simulink model "LQR"  (R2018a)
settings: Solver=ode45  StartTime=0.0  StopTime=10.0  RelTol=1e-3  EnableMultiTasking=on
values from neighbouring files (symbols this model uses):
  A = input('enter the A matrix = ')    [LQR2.m]
  B = input('enter the B matrix = ')    [LQR2.m]
  Q = transpose(C)*C    [LQR2.m]
  R = input('enter the matrix of R(no. of columns must be equal to B) = ')    [LQR2.m]
undefined symbols (not defined in the file or in its folder): X0
libraries: dspinverses x1
settings Model: Creator=gkavuran  LastModifiedBy=Jay
settings DataIOCC: LimitDataPoints=on  SaveFormat=Array
settings OptimizationCC: LifeSpan=inf
settings DebuggingCC: SolverPrmCheckMsg=warning  SFUnexpectedBacktrackingDiag=warning  SFNoUnconditionalDefaultTransitionDiag=warning  SFExecutionAtInitializationDiag=none
settings HardwareCC: ProdBitPerPointer=32  ProdBitPerSizeT=32  ProdBitPerPtrDiffT=32  ProdLargestAtomicFloat=None  ProdIntDivRoundTo=Undefined  ProdEndianess=Unspecified  ProdWordSize=32  ProdHWDeviceType=32-bit Generic
settings ModelReferenceCC: PropagateSignalLabelsOutOfModel=off
settings CodeAppCC: StateflowObjectComments=on
settings GRTTargetCC: TargetLangStandard=C89/C90 (ANSI)  GeneratePreprocessorConditionals=Disable all
settings ConfigComp: CovMetricSettings=dw  CovHtmlReporting=on  CovSaveCumulativeToWorkspaceVar=on  CovSaveSingleToWorkspaceVar=on  CovExternalEMLEnable=off  CovSFcnEnable=off

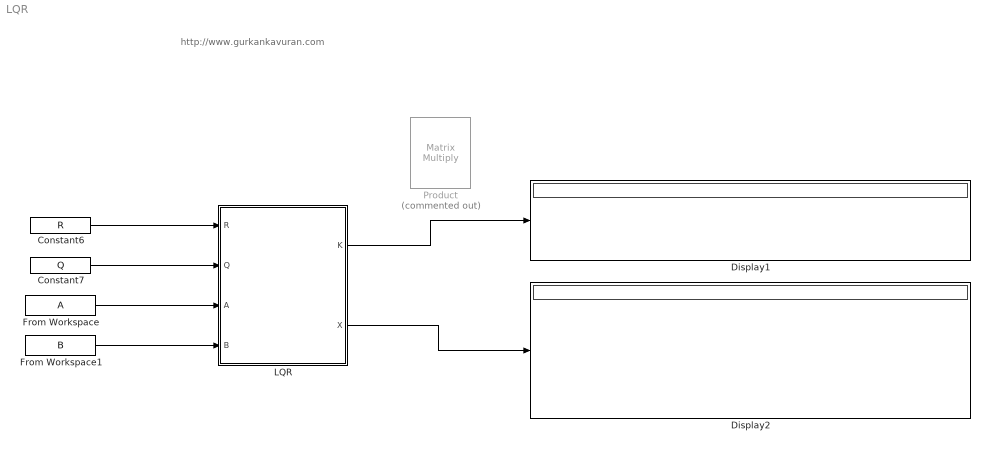
== system LQR ==
  note: http://www.gurkankavuran.com
  Constant6 : Constant  Value=R
  Constant7 : Constant  Value=Q
  Display1 : Display
  Display2 : Display
  From Workspace : FromWorkspace  VariableName=A  SampleTime=0
  From Workspace1 : FromWorkspace  VariableName=B  SampleTime=0
  LQR : Subsystem  Description=|  TreatAsAtomicUnit=on  mask(LQR with Algebric Riccati Equation){A=A, B=B, X0=X0}
      | LQR Block
      | 
      | by Gurkan KAVURAN
      | gurkankavuran@gmail.com
      mask prompts: A "A (System Matrix)"; B "B (System Matrix)"; X0 "Xo (Initial Values of States)"
      mask help:
      | It is easy to optimize Q and R matrices with online process.
      | Please see the help file to define the block parameters.
      mask Help:
      | Parameters Example:
      | 
      | Q = diag([500 1 1 0 1 1] );
      | R = 1*diag([0.01 0.01 0.01 0.01]);
      | X0=[0 0 0 0 0 0;0 0 0 0 0 0;0 0 0 0 0 0;0 0 0 0 0 0;0 0 0 0 0 0;0 0 0 0 0 0];
      | 
      | "Matrix multiply" block is recommended to use in state feedback control mechanism.
      | 
      | 
      | http://www.gurkankavuran.com
      mask Display:
      | disp('LQR')
      | port_label('input', 1, 'R')
      | port_label('input', 2, 'Q')
      | port_label('output', 1, 'K')
      | port_label('output', 2, 'X')
  Product : Product  Commented=on  Multiplication=Matrix(*)
  wires:
  LQR/1(K) -> Display1/1
  Constant6/1 -> LQR/1(R)
  Constant7/1 -> LQR/2(Q)
  LQR/2(X) -> Display2/1
  From Workspace/1 -> LQR/3(A)
  From Workspace1/1 -> LQR/4(B)

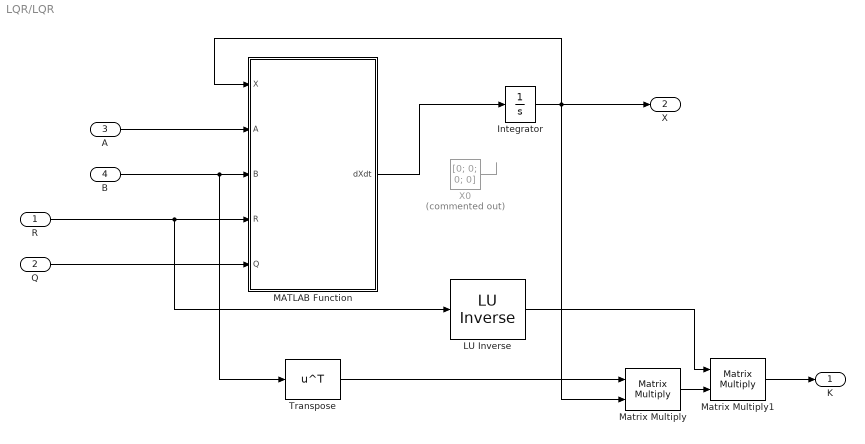
== system LQR/LQR ==
  R : Inport
  Q : Inport  Port=2
  A : Inport  Port=3
  B : Inport  Port=4
  " LU Inverse" : dspinverses/ LU Inverse
      settings: SourceProductName=DSP System Toolbox
  Integrator : Integrator  InitialCondition=[0; 0; 0; 0]
  MATLAB Function : MATLAB Function  TreatAsAtomicUnit=on
  Matrix Multiply : Product  Multiplication=Matrix(*)
  Matrix Multiply1 : Product  Multiplication=Matrix(*)
  Transpose : Math  Operator=transpose  SaturateOnIntegerOverflow=on
  X0 : Constant  Commented=on  Value=[0; 0; 0; 0]
  K : Outport
  X : Outport  Port=2
  wires:
  Matrix Multiply1/1 -> K/1
  A/1 -> MATLAB Function/2(A)
  B/1 -> Transpose/1, MATLAB Function/3(B)
  " LU Inverse"/1 -> Matrix Multiply1/1
  X0/1 -> ?
  Matrix Multiply/1 -> Matrix Multiply1/2
  Transpose/1 -> Matrix Multiply/1
  MATLAB Function/1(dXdt) -> Integrator/1
  Integrator/1 -> X/1, Matrix Multiply/2, MATLAB Function/1(X)
  Q/1 -> MATLAB Function/5(Q)
  R/1 -> " LU Inverse"/1, MATLAB Function/4(R)

== matlab function LQR/MATLAB Function ==
  data: dXdt output; X input; A input; B input; R input; Q input
function dXdt  = mRiccati(X, A, B,R,Q)

X = reshape(X, size(A)); %Convert from "n^2"-by-1 to "n"-by-"n"

%Determine derivative
dXdt = A.'*X + X*A - (X*B)/(R)*(B.'*X) + Q; %inv(R) is slow 

% dXdtS= dXdt(:); %Convert from "n"-by-"n" to "n^2"-by-1,algebraic Riccati equation (ARE)
